simulink model "TemplateNIPID"  (Simulink 7.3)
settings: Solver=ode5  StartTime=0.0  StopTime=inf  FixedStep=0.1  RelTol=1e-3
undefined symbols (not defined in the file): eta1_0_real, v1_0_real, velocitySatValues1
libraries: simulink x41, dspmtrx3 x16, marine_gnc x6, dspindex x5, simulink_extras x1, dspinverses x1
(part 3 of 4)

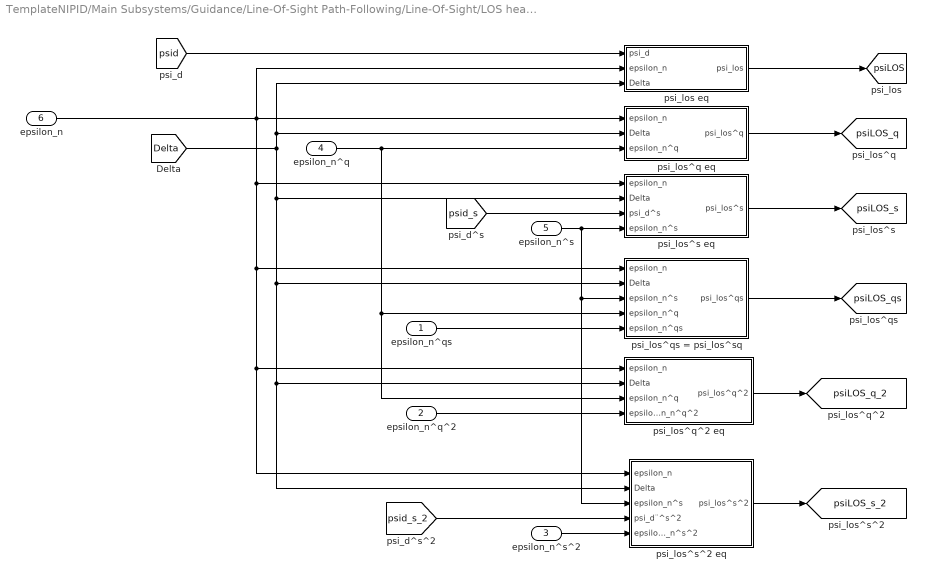
== system TemplateNIPID/Main Subsystems/Guidance/Line-Of-Sight Path-Following/Line-Of-Sight/LOS heading ==
  epsilon_n^qs : Inport
  epsilon_n^q^2 : Inport  Port=2
  epsilon_n^s^2 : Inport  Port=3
  epsilon_n^q : Inport  Port=4
  epsilon_n^s : Inport  Port=5
  epsilon_n : Inport  Port=6
  psi_los eq : Subsystem
  psi_los^q eq : Subsystem
  psi_los^q^2 eq : Subsystem
  psi_los^qs = psi_los^sq : Subsystem
  psi_los^s eq : Subsystem
  psi_los^s^2 eq : Subsystem
  tag scope: psiLOS=global, psiLOS_q=global, psiLOS_q_2=global, psiLOS_qs=global, psiLOS_s=global, psiLOS_s_2=global
  wires:
  psi_los^s^2 eq/1(psi_los^s^2) -> [psiLOS_s_2]
  epsilon_n^s^2/1 -> psi_los^s^2 eq/5(epsilon_n^s^2)
  [psid_s_2] -> psi_los^s^2 eq/4(psi_d¨^s^2)
  epsilon_n^q^2/1 -> psi_los^q^2 eq/4(epsilon_n^q^2)
  psi_los^q^2 eq/1(psi_los^q^2) -> [psiLOS_q_2]
  epsilon_n^qs/1 -> psi_los^qs = psi_los^sq/5(epsilon_n^qs)
  epsilon_n^s/1 -> psi_los^s eq/4(epsilon_n^s), psi_los^s^2 eq/3(epsilon_n^s), psi_los^qs = psi_los^sq/3(epsilon_n^s)
  psi_los^qs = psi_los^sq/1(psi_los^qs) -> [psiLOS_qs]
  [psid_s] -> psi_los^s eq/3(psi_d^s)
  psi_los^s eq/1(psi_los^s) -> [psiLOS_s]
  psi_los^q eq/1(psi_los^q) -> [psiLOS_q]
  epsilon_n^q/1 -> psi_los^q eq/3(epsilon_n^q), psi_los^q^2 eq/3(epsilon_n^q), psi_los^qs = psi_los^sq/4(epsilon_n^q)
  [Delta] -> psi_los^q eq/2(Delta), psi_los^s eq/2(Delta), psi_los^qs = psi_los^sq/2(Delta), psi_los^s^2 eq/2(Delta), psi_los^q^2 eq/2(Delta), psi_los eq/3(Delta)
  epsilon_n/1 -> psi_los^q eq/1(epsilon_n), psi_los^s eq/1(epsilon_n), psi_los^qs = psi_los^sq/1(epsilon_n), psi_los^s^2 eq/1(epsilon_n), psi_los^q^2 eq/1(epsilon_n), psi_los eq/2(epsilon_n)
  [psid] -> psi_los eq/1(psi_d)
  psi_los eq/1(psi_los) -> [psiLOS]

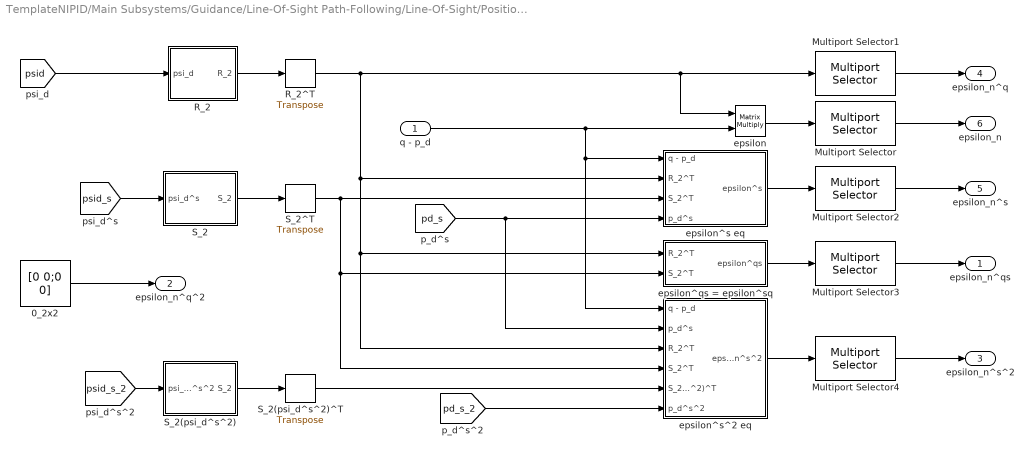
== system TemplateNIPID/Main Subsystems/Guidance/Line-Of-Sight Path-Following/Line-Of-Sight/Position error signals ==
  q - p_d : Inport  OutDataType=fixdt(1, 16)  OutScaling=2^0
  0_2x2 : Constant  Value=[0 0;0 0]  OutDataType=fixdt(1, 16)  OutScaling=2^0
  Multiport Selector{,1..4} (5 alike) : dspindex/Multiport Selector  rowsOrCols=Rows  idxCellArray={2}  idxErrMode=Clip Index
  R_2 : Subsystem  TreatAsAtomicUnit=on
      settings: MinAlgLoopOccurrences=on
  R_2^T : dspmtrx3/Transpose  SystemSampleTime=-1  Hermitian=off  overflowFlag=off
  S_2 : Subsystem  TreatAsAtomicUnit=on
      settings: MinAlgLoopOccurrences=on
  S_2(psi_d^s^2) : Subsystem  TreatAsAtomicUnit=on
      settings: MinAlgLoopOccurrences=on
  S_2(psi_d^s^2)^T : dspmtrx3/Transpose  SystemSampleTime=-1  Hermitian=off  overflowFlag=off
  S_2^T : dspmtrx3/Transpose  SystemSampleTime=-1  Hermitian=off  overflowFlag=off
  epsilon : Product  Multiplication=Matrix(*)  OutDataType=fixdt(1, 16)  OutScaling=2^0  RndMeth=Zero
  epsilon^qs = epsilon^sq : Subsystem
  epsilon^s eq : Subsystem
  epsilon^s^2 eq : Subsystem
  epsilon_n^qs : Outport
  epsilon_n^q^2 : Outport  Port=2
  epsilon_n^s^2 : Outport  Port=3
  epsilon_n^q : Outport  Port=4
  epsilon_n^s : Outport  Port=5
  epsilon_n : Outport  Port=6
  wires:
  Multiport Selector1/1 -> epsilon_n^q/1
  [pd_s_2] -> epsilon^s^2 eq/6(p_d^s^2)
  S_2(psi_d^s^2)^T/1 -> epsilon^s^2 eq/5(S_2(psi_d^s^2)^T)
  Multiport Selector4/1 -> epsilon_n^s^2/1
  epsilon^s^2 eq/1(epsilon^s^2) -> Multiport Selector4/1
  S_2(psi_d^s^2)/1(S_2) -> S_2(psi_d^s^2)^T/1
  Multiport Selector3/1 -> epsilon_n^qs/1
  Multiport Selector2/1 -> epsilon_n^s/1
  Multiport Selector/1 -> epsilon_n/1
  epsilon/1 -> Multiport Selector/1
  0_2x2/1 -> epsilon_n^q^2/1
  epsilon^qs = epsilon^sq/1(epsilon^qs) -> Multiport Selector3/1
  S_2^T/1 -> epsilon^s^2 eq/4(S_2^T), epsilon^qs = epsilon^sq/2(S_2^T), epsilon^s eq/3(S_2^T)
  epsilon^s eq/1(epsilon^s) -> Multiport Selector2/1
  [pd_s] -> epsilon^s^2 eq/2(p_d^s), epsilon^s eq/4(p_d^s)
  S_2/1(S_2) -> S_2^T/1
  q - p_d/1 -> epsilon^s^2 eq/1(q - p_d), epsilon^s eq/1(q - p_d), epsilon/2
  R_2^T/1 -> epsilon^s^2 eq/3(R_2^T), epsilon^qs = epsilon^sq/1(R_2^T), epsilon^s eq/2(R_2^T), Multiport Selector1/1, epsilon/1
  [psid] -> R_2/1(psi_d)
  R_2/1(R_2) -> R_2^T/1
  [psid_s] -> S_2/1(psi_d^s)
  [psid_s_2] -> S_2(psi_d^s^2)/1(psi_d^s^2)

== system TemplateNIPID/Main Subsystems/Guidance/Line-Of-Sight Path-Following/Line-Of-Sight/Virtual Vessel ==
  0_2x1 : Constant  Value=[0;0]  VectorParams1D=off  OutDataType=fixdt(1, 16)  OutScaling=2^0
  I : dspmtrx3/Constant Diagonal Matrix  SystemSampleTime=-1  q=[1 1]  frame=off  dataType=Inherit from 'Constant(s) along diagonal'  isSigned=on  wordLen=16  udDataType=sfix(16)  fracBitsMode=Best precision  numFracBits=15
  Matrix Concatenate : Concatenate  Mode=Multidimensional array
  Vector Concatenate : Concatenate  Mode=Vector
  Vector Concatenate1 : Concatenate  Mode=Vector
  tag scope: chi=global, chi_q=global, chi_s=global
  wires:
  0_2x1/1 -> Vector Concatenate1/1
  Vector Concatenate1/1 -> [chi_s]
  Matrix Concatenate/1 -> [chi_q]
  [psiLOS_q] -> Matrix Concatenate/2
  I/1 -> Matrix Concatenate/1
  Vector Concatenate/1 -> [chi]
  [psiLOS] -> Vector Concatenate/2
  [q] -> Vector Concatenate/1
  [psiLOS_s] -> Vector Concatenate1/2

== system TemplateNIPID/Main Subsystems/Guidance/Line-Of-Sight Path-Following/Path/Ellipse path ==
  p_d eq : Subsystem
  p_d^s eq : Subsystem
  p_d^s^2 eq : Subsystem
  p_d^s^3 eq : Subsystem
  |p_d^s| eq : Subsystem
  tag scope: pdEllipse=global, pd_sEllipse=global, pd_s_2Ellipse=global, pd_s_3Ellipse=global, pd_sabsEllipse=global
  wires:
  p_d^s eq/1(p_d^s) -> [pd_sEllipse], |p_d^s| eq/1(p_d^s)
  [s] -> p_d eq/1(s), p_d^s eq/1(s), p_d^s^2 eq/1(s), p_d^s^3 eq/1(s)
  [rx] -> p_d eq/2(r_x), p_d^s eq/2(r_x), p_d^s^2 eq/2(r_x), p_d^s^3 eq/2(r_x)
  [ry] -> p_d eq/3(r_y), p_d^s eq/3(r_y), p_d^s^2 eq/3(r_y), p_d^s^3 eq/3(r_y)
  [x0] -> p_d eq/4(origo_x)
  [y0] -> p_d eq/5(origo_y)
  [k] -> p_d eq/6(k), p_d^s eq/4(k), p_d^s^2 eq/4(k), p_d^s^3 eq/4(k)
  p_d eq/1(p_d) -> [pdEllipse]
  |p_d^s| eq/1(|p_d^s|) -> [pd_sabsEllipse]
  p_d^s^2 eq/1(p_d^s^2) -> [pd_s_2Ellipse]
  p_d^s^3 eq/1(p_d^s^3) -> [pd_s_3Ellipse]

== system TemplateNIPID/Main Subsystems/Guidance/Line-Of-Sight Path-Following/Path/Path Switch workaround + limiter ==
  note: Path Selector == 1: Linear path
      | Path Selector == 0: Ellipse path
  Limiter : Subsystem
  Rounding Function : Rounding
  Saturation : Saturate  UpperLimit=1  LowerLimit=0  OutDataType=fixdt(1, 16)  OutScaling=2^0
  p_d selcetor : Subsystem
  p_d^s selcetor : Subsystem
  p_d^s^2 selcetor : Subsystem
  p_d^s^3 selcetor : Subsystem
  p_d^s^3 selcetor1 : Subsystem
  tag scope: pd=global, pd_s=global, pd_s_2=global, pd_s_3=global, pd_sabs=global
  wires:
  [pathSelector] -> Saturation/1  "chosen path"
  p_d selcetor/1(p_d) -> Limiter/1(p_d)
  Limiter/1(sat_p_d) -> [pd]
  p_d^s selcetor/1(p_d^s) -> [pd_s]
  p_d^s^2 selcetor/1(p_d^s^2) -> [pd_s_2]
  p_d^s^3 selcetor/1(p_d^s^3) -> [pd_s_3]
  p_d^s^3 selcetor1/1(|p_d^s|) -> [pd_sabs]
  Rounding Function/1 -> p_d selcetor/1(Path Selector), p_d^s selcetor/1(Path Selector), p_d^s^2 selcetor/1(Path Selector), p_d^s^3 selcetor/1(Path Selector), p_d^s^3 selcetor1/1(Path Selector)
  Saturation/1 -> Rounding Function/1

== system TemplateNIPID/Main Subsystems/Guidance/Line-Of-Sight Path-Following/Path/Straight path ==
  0_2x1 : Constant  Value=[0;0]  VectorParams1D=off  OutDataType=fixdt(1, 16)  OutScaling=2^0
  p_d eq : Subsystem
  p_d^s eq : Subsystem
  |p_d^s| eq : Subsystem
  tag scope: pdLinear=global, pd_sLinear=global, pd_s_2Linear=global, pd_s_3Linear=global, pd_sabsLinear=global
  wires:
  p_d eq/1(p_d) -> [pdLinear]
  0_2x1/1 -> [pd_s_2Linear], [pd_s_3Linear]
  [y2] -> p_d eq/5(y_2), p_d^s eq/4(y_2)
  [x2] -> p_d eq/4(x_2), p_d^s eq/3(x_2)
  [y1] -> p_d eq/3(y_1), p_d^s eq/2(y_1)
  [x1] -> p_d eq/2(x_1), p_d^s eq/1(x_1)
  [s] -> p_d eq/1(s)
  |p_d^s| eq/1(|p_d^s|) -> [pd_sabsLinear]
  p_d^s eq/1(p_d^s) -> |p_d^s| eq/1(p_d^s), [pd_sLinear]

== system TemplateNIPID/Main Subsystems/Guidance/Line-Of-Sight Path-Following/Speed assigment/v_s eq ==
  |p_d^s| : Inport
  u_d : Inport  Port=2
  Divide : Product  Inputs=*/  OutDataType=fixdt(1, 16)  OutScaling=2^-10
  v_s : Outport
  wires:
  |p_d^s|/1 -> Divide/2
  u_d/1 -> Divide/1
  Divide/1 -> v_s/1

== system TemplateNIPID/Main Subsystems/Guidance/Line-Of-Sight Path-Following/Speed assigment/v_s^s eq ==
  |p_d^s| : Inport
  u_d : Inport  Port=2
  p_d^s : Inport  Port=3
  p_d^s^2 : Inport  Port=4
  Constant : Constant  Value=3  OutDataType=fixdt(1, 16)  OutScaling=2^0
  Divide : Product  Inputs=*/  OutDataType=fixdt(1, 16)  OutScaling=2^-10
  Gain : Gain  Gain=-1  ParameterDataType=fixdt(1, 16)  ParameterScaling=2^0  OutDataType=fixdt(1, 16)  OutScaling=2^0
  Product : Product  OutDataType=fixdt(1, 16)  OutScaling=2^0  RndMeth=Zero
  Product1 : Product  Multiplication=Matrix(*)  OutDataType=fixdt(1, 16)  OutScaling=2^0  RndMeth=Zero
  p_d^s^T : dspmtrx3/Transpose  SystemSampleTime=-1  Hermitian=off  overflowFlag=off
  |p_d^s|^3 : Math  Operator=pow  OutDataType=fixdt(1, 16)  OutScaling=2^0  SaturateOnIntegerOverflow=on
  v_s^s : Outport
  wires:
  Gain/1 -> v_s^s/1
  u_d/1 -> Product/2
  Divide/1 -> Product/1
  |p_d^s|^3/1 -> Divide/2
  Product1/1 -> Divide/1
  Constant/1 -> |p_d^s|^3/2
  |p_d^s|/1 -> |p_d^s|^3/1
  p_d^s^2/1 -> Product1/2
  p_d^s^T/1 -> Product1/1
  p_d^s/1 -> p_d^s^T/1
  Product/1 -> Gain/1

== system TemplateNIPID/Main Subsystems/Guidance/Line-Of-Sight Path-Following/Speed assigment/v_s^t eq ==
  |p_d^s| : Inport
  u_d^t : Inport  Port=2
  Divide : Product  Inputs=*/  OutDataType=fixdt(1, 16)  OutScaling=2^-10
  v_s^t : Outport
  wires:
  |p_d^s|/1 -> Divide/2
  u_d^t/1 -> Divide/1
  Divide/1 -> v_s^t/1

== system TemplateNIPID/Main Subsystems/Naviagation/Input from SIT/u_act to tau/u_act to f_act ==
  u_act : Inport
  Demux : Demux  Outputs=5
  Mux : Mux  Inputs=5
  u_1 to f_1 VSP speed 0.3 : Subsystem
  u_2 to f_2 VSP speed 0.3 : Subsystem
  u_3 to f_3 VSP speed 0.3 : Subsystem
  u_4 to f_4 VSP speed 0.3 : Subsystem
  u_5 to f_5 BT power 0.4 : Subsystem
  f_act : Outport
  wires:
  Demux/2 -> u_2 to f_2 VSP speed 0.3/1(u_2)
  u_act/1 -> Demux/1
  Mux/1 -> f_act/1
  Demux/1 -> u_1 to f_1 VSP speed 0.3/1(u_1)
  Demux/3 -> u_3 to f_3 VSP speed 0.3/1(u_3)
  Demux/4 -> u_4 to f_4 VSP speed 0.3/1(u_4)
  Demux/5 -> u_5 to f_5 BT power 0.4/1(u_5)
  u_1 to f_1 VSP speed 0.3/1(f_1) -> Mux/1
  u_2 to f_2 VSP speed 0.3/1(f_2) -> Mux/2
  u_3 to f_3 VSP speed 0.3/1(f_3) -> Mux/3
  u_4 to f_4 VSP speed 0.3/1(f_4) -> Mux/4
  u_5 to f_5 BT power 0.4/1(f_5) -> Mux/5

== system TemplateNIPID/Main Subsystems/Plant/Linear Simulator/Linear Vessel Dynamics/R(psi) ==
  psi : Inport
  Mux : Mux  Inputs=9
  R(psi) : Reshape  OutputDimensionality=Customize  OutputDimensions=[3,3]
  R11 : Fcn  Expr=cos(u(1))
  R12 : Fcn  Expr=-1*sin(u(1))
  R{13,23,31..32} (4 alike) : Constant  Value=0
  R21 : Fcn  Expr=sin(u(1))
  R22 : Fcn  Expr=cos(u(1))
  R33 : Constant
  R : Outport
  wires:
  R(psi)/1 -> R/1
  Mux/1 -> R(psi)/1
  psi/1 -> R11/1, R21/1, R12/1, R22/1
  R11/1 -> Mux/1
  R21/1 -> Mux/2
  R31/1 -> Mux/3
  R12/1 -> Mux/4
  R22/1 -> Mux/5
  R32/1 -> Mux/6
  R13/1 -> Mux/7
  R33/1 -> Mux/9
  R23/1 -> Mux/8

== system TemplateNIPID/Main Subsystems/Control/Nonlinear PID/Control law/tau_FF/S(r)^T ==
  Mux : Mux  Inputs=9
  R31 : Constant  Value=0
  S(r) : Reshape  OutputDimensionality=Customize  OutputDimensions=[3,3]
  S{11,13,22..23,32} (5 alike) : Constant  Value=0
  S12 : Gain  ParameterDataType=fixdt(1, 16)  ParameterScaling=2^0  OutDataType=fixdt(1, 16)  OutScaling=2^0
  S33 : Constant
  S^T : dspmtrx3/Transpose  SystemSampleTime=-1  Hermitian=off  overflowFlag=off
  r : Selector  InputPortWidth=3  IndexOptions=Index vector (dialog)  Indices=[3]  OutputSizes=1
  S(r)^T : Outport
  wires:
  S(r)/1 -> S^T/1
  Mux/1 -> S(r)/1
  R31/1 -> Mux/3
  S12/1 -> Mux/4
  S22/1 -> Mux/5
  S32/1 -> Mux/6
  S13/1 -> Mux/7
  S33/1 -> Mux/9
  S23/1 -> Mux/8
  S11/1 -> Mux/1
  r/1 -> Mux/2, S12/1
  [nu] -> r/1
  S^T/1 -> S(r)^T/1

== system TemplateNIPID/Main Subsystems/Control/Nonlinear PID/e_1/Heading to -pi/pi/rad to [-pi pi] ==
  rad : Inport  OutDataType=sfix(16)  OutScaling=2^0
  Constant : Constant  Value=2*pi  OutDataType=sfix(16)  OutScaling=2^0
  Gain : Gain  Gain=pi  ParameterDataType=sfix(16)  ParameterScaling=2^0  OutDataType=sfix(16)  OutScaling=2^0  SaturateOnIntegerOverflow=on  OutDataTypeStr=Inherit: Same as input  ParamDataTypeStr=Inherit: Same as input
  Math Function : Math  Operator=rem  OutDataType=sfix(16)  OutScaling=2^0  SaturateOnIntegerOverflow=on
  Saturation : Saturate  UpperLimit=1e10  LowerLimit=-1e10
  Sign : Signum
  Sum : Sum  Inputs=|+-  OutDataType=sfix(16)  OutScaling=2^0  SaturateOnIntegerOverflow=on
  Sum1 : Sum  Inputs=|++  OutDataType=sfix(16)  OutScaling=2^0  SaturateOnIntegerOverflow=on
  "[-pi pi]" : Outport  OutDataType=sfix(16)  OutScaling=2^0
  wires:
  Sum/1 -> "[-pi pi]"/1
  Math Function/1 -> Sum/1
  Constant/1 -> Math Function/2
  Sum1/1 -> Math Function/1
  Gain/1 -> Sum1/2, Sum/2
  Sign/1 -> Gain/1
  rad/1 -> Saturation/1
  Saturation/1 -> Sign/1, Sum1/1

== system TemplateNIPID/Main Subsystems/Control/Nonlinear PID/e_1/Heading to -pi/pi1/rad to [-pi pi] ==
  rad : Inport  OutDataType=sfix(16)  OutScaling=2^0
  Constant : Constant  Value=2*pi  OutDataType=sfix(16)  OutScaling=2^0
  Gain : Gain  Gain=pi  ParameterDataType=sfix(16)  ParameterScaling=2^0  OutDataType=sfix(16)  OutScaling=2^0  SaturateOnIntegerOverflow=on  OutDataTypeStr=Inherit: Same as input  ParamDataTypeStr=Inherit: Same as input
  Math Function : Math  Operator=rem  OutDataType=sfix(16)  OutScaling=2^0  SaturateOnIntegerOverflow=on
  Saturation : Saturate  UpperLimit=1e10  LowerLimit=-1e10
  Sign : Signum
  Sum : Sum  Inputs=|+-  OutDataType=sfix(16)  OutScaling=2^0  SaturateOnIntegerOverflow=on
  Sum1 : Sum  Inputs=|++  OutDataType=sfix(16)  OutScaling=2^0  SaturateOnIntegerOverflow=on
  "[-pi pi]" : Outport  OutDataType=sfix(16)  OutScaling=2^0
  wires:
  Sum/1 -> "[-pi pi]"/1
  Math Function/1 -> Sum/1
  Constant/1 -> Math Function/2
  Sum1/1 -> Math Function/1
  Gain/1 -> Sum1/2, Sum/2
  Sign/1 -> Gain/1
  rad/1 -> Saturation/1
  Saturation/1 -> Sign/1, Sum1/1

== system TemplateNIPID/Main Subsystems/Control/PS3 u input control/u_act to tau/u_act to f_act/u_1 to f_1 VSP speed 0.3 ==
  note: Table valid for VSP speed == 0.30
  u_1 : Inport
  u_1 to f_1 : Lookup  InputValues=[-1.0000 -0.9500 -0.9000 -0.8500 -0.8000 -0.7500 -0.7000 -0.6500 -0.6000 -0.5500 -0.5000 -0.4500 -0.4000 -0.3500 -0.3000 -0.2500 -0.2000 -0.1500 -0.1000 -0.0500 0 0.0500 0.1000 0.1500 0.2000 0.2500 0.3000 0.3500 0.4000 0.4500 0.5000 0.5500 0.6000 0.6500 0.7000 0.7500 0.8000 0.8500 0.9000]  Table=[-0.6829 -0.6369 -0.5785 -0.5165 -0.4456 -0.3725 -0.3308 -0.2827 -0.2277 -0.1517 -0.1240 -0.0769 -0.0238 0.0039 0.0377 0.0635 0.1051 0.1196 0.1412 0.1721 0.1754 0.1774 0.2104 0.2200 0.2266 0.2673 0.3025 0.3486 0.3896 0.4252 0.4782 0.5164 0.5695 0.6195 0.6723 0.7449 0.7836 0.8414 0.8987 ]  LookUpMeth=Interpolation-Use End Values  OutDataType=fixdt(1, 16)  OutScaling=2^0
  f_1 : Outport
  wires:
  u_1/1 -> u_1 to f_1/1
  u_1 to f_1/1 -> f_1/1

== system TemplateNIPID/Main Subsystems/Control/PS3 u input control/u_act to tau/u_act to f_act/u_2 to f_2 VSP speed 0.3 ==
  note: Switching to the lookup table giving the closes value
  note: workaround setup
  note: Tables valid for VSP speed == 0.30
  u_2 : Inport
  Gain1 : Gain  Gain=3  ParameterDataType=fixdt(1, 16)  ParameterScaling=2^0  OutDataType=fixdt(1, 16)  OutScaling=2^0
  If < 0.00391 : simulink/Logic and Bit Operations/Compare To Constant  SystemSampleTime=-1  relop=<  const=-0.5  LogicOutDataTypeMode=uint8
  If < 0.06731 : simulink/Logic and Bit Operations/Compare To Constant  SystemSampleTime=-1  relop=<  const=-0.1  LogicOutDataTypeMode=uint8
  If >= 0.00391 : simulink/Logic and Bit Operations/Compare To Constant  SystemSampleTime=-1  relop=>=  const=-0.5  LogicOutDataTypeMode=uint8
  If >= 0.06731 : simulink/Logic and Bit Operations/Compare To Constant  SystemSampleTime=-1  relop=>=  const=-0.1  LogicOutDataTypeMode=uint8
  Logical Operator : Logic  AllPortsSameDT=off  OutDataTypeMode=boolean  LogicDataType=fixdt(0, 8)  OutDataTypeStr=boolean
  Multiport Switch : MultiPortSwitch  OutDataType=fixdt(1, 16)  OutScaling=2^0
  Sum : Sum  Inputs=+++  OutDataType=fixdt(1, 16)  OutScaling=2^0
  Sum1 : Sum  Inputs=|++  OutDataType=fixdt(1, 16)  OutScaling=2^0
  u_2 < -0.1 && u_2 >= -0.2 : Lookup  InputValues=|  Table=|  LookUpMeth=Interpolation-Use End Values  OutDataType=fixdt(1, 16)  OutScaling=2^0
      InputValues=|
      | [-0.2000
      |    -0.1500
      |    -0.1000]
      Table=|
      | [-0.0105
      |     0.0226
      |     0.0673]
  u_2 < -0.5 : Lookup  InputValues=|  Table=|  LookUpMeth=Interpolation-Use End Values  OutDataType=fixdt(1, 16)  OutScaling=2^0
      InputValues=|
      | [-1.0000
      |    -0.9500
      |    -0.9000
      |    -0.8500
      |    -0.8000
      |    -0.7500
      |    -0.7000
      |    -0.6500
      |    -0.6000
      |    -0.5500
      |    -0.5000]
      Table=|
      | [-0.2704
      |    -0.2259
      |    -0.1903
      |    -0.1697
      |    -0.1518
      |    -0.1234
      |    -0.0994
      |    -0.0817
      |    -0.0612
      |    -0.0123
      |     0.0039]
  u_2 => 0 : Lookup  InputValues=|  Table=|  LookUpMeth=Interpolation-Use End Values  OutDataType=fixdt(1, 16)  OutScaling=2^0
      InputValues=|
      | [0
      |     0.0500
      |     0.1000
      |     0.1500
      |     0.2000
      |     0.2500
      |     0.3000
      |     0.3500
      |     0.4000
      |     0.4500
      |     0.5000
      |     0.5500
      |     0.6000
      |     0.6500
      |     0.7000
      |     0.7500
      |     0.8000
      |     0.8500]
      Table=|
      | [0.0872
      |     0.0930
      |     0.1182
      |     0.1412
      |     0.1892
      |     0.2146
      |     0.2678
      |     0.3096
      |     0.3551
      |     0.4013
      |     0.4566
      |     0.5051
      |     0.5477
      |     0.6060
      |     0.6703
      |     0.7437
      |     0.7604
      |     0.7634]
  f_2 : Outport
  wires:
  Multiport Switch/1 -> f_2/1
  Sum/1 -> Multiport Switch/1
  If >= 0.06731/1 -> Gain1/1
  If < 0.00391/1 -> Sum/1
  u_2/1 -> u_2 < -0.5/1, If >= 0.06731/1, If < 0.00391/1, If >= 0.00391/1, If < 0.06731/1, u_2 => 0/1, u_2 < -0.1 && u_2 >= -0.2/1
  u_2 < -0.5/1 -> Multiport Switch/2
  u_2 => 0/1 -> Multiport Switch/4
  u_2 < -0.1 && u_2 >= -0.2/1 -> Multiport Switch/3
  If < 0.06731/1 -> Logical Operator/2
  If >= 0.00391/1 -> Logical Operator/1
  Gain1/1 -> Sum/3
  Sum1/1 -> Sum/2
  Logical Operator/1 -> Sum1/1, Sum1/2

== system TemplateNIPID/Main Subsystems/Control/PS3 u input control/u_act to tau/u_act to f_act/u_3 to f_3 VSP speed 0.3 ==
  note: Table valid for VSP speed == 0.30
  u_3 : Inport
  u_3 to f_3 : Lookup  InputValues=[-1.0000,-0.9500,-0.9000,-0.8500,-0.8000,-0.7500,-0.7000,-0.6500,-0.6000,-0.5500,-0.5000,-0.4500,-0.4000,-0.3500,-0.3000,-0.2000,-0.1500,-0.1000,-0.0500,0,0.0500,0.1000,0.1500,0.2000,0.2500,0.3000,0.3500,0.4000,0.4500,0.5000,0.5500,0.6000,0.6500,0.7000,0.7500,0.8000,0.8500,0.9500,1.0000]  Table=[-0.5408,-0.5036,-0.4487,-0.3802,-0.3147,-0.2525,-0.2338,-0.1568,-0.1034,-0.0647,-0.0054,0.0221,0.0572,0.0747,0.0991,0.1258,0.1385,0.1447,0.1539,0.1625,0.1712,0.1976,0.2258,0.2443,0.3058,0.3460,0.3989,0.4342,0.4932,0.5524,0.5814,0.6394,0.6851,0.7496,0.8081,0.8382,0.8665,0.8767,0.8885]  LookUpMeth=Interpolation-Use End Values  OutDataType=fixdt(1, 16)  OutScaling=2^0
  f_3 : Outport
  wires:
  u_3/1 -> u_3 to f_3/1
  u_3 to f_3/1 -> f_3/1

== system TemplateNIPID/Main Subsystems/Control/PS3 u input control/u_act to tau/u_act to f_act/u_4 to f_4 VSP speed 0.3 ==
  note: Tables valid for VSP speed == 0.30
  u_4 : Inport
  Gain : Gain  Gain=2  ParameterDataType=fixdt(1, 16)  ParameterScaling=2^0  OutDataType=fixdt(1, 16)  OutScaling=2^0
  If < 0.0451 : simulink/Logic and Bit Operations/Compare To Constant  SystemSampleTime=-1  relop=<  const=-0.1  LogicOutDataTypeMode=uint8
  If >= 0.0451 : simulink/Logic and Bit Operations/Compare To Constant  SystemSampleTime=-1  relop=>=  const=-0.1  LogicOutDataTypeMode=uint8
  Multiport Switch : MultiPortSwitch  Inputs=2  OutDataType=fixdt(1, 16)  OutScaling=2^0
  Sum : Sum  Inputs=+|+  OutDataType=fixdt(1, 16)  OutScaling=2^0
  u_4 < -0.1 : Lookup  InputValues=|  Table=|  LookUpMeth=Interpolation-Use End Values  OutDataType=fixdt(1, 16)  OutScaling=2^0
      InputValues=|
      | [-0.8000
      |    -0.7500
      |    -0.7000
      |    -0.6500
      |    -0.6000
      |    -0.5500
      |    -0.5000
      |    -0.4500
      |    -0.4000
      |    -0.3500
      |    -0.3000
      |    -0.2500
      |    -0.2000
      |    -0.1500
      |    -0.1000]
      Table=|
      | [-0.5212
      |    -0.5163
      |    -0.4943
      |    -0.4390
      |    -0.3803
      |    -0.3603
      |    -0.3132
      |    -0.2567
      |    -0.2102
      |    -0.1609
      |    -0.1267
      |    -0.0819
      |    -0.0554
      |     0.0099
      |     0.0450]
  u_4 >= -0.1 : Lookup  InputValues=|  Table=|  LookUpMeth=Interpolation-Use End Values  OutDataType=fixdt(1, 16)  OutScaling=2^0
      InputValues=|
      | [0.0431
      |     0.0808
      |     0.0867
      |     0.1337
      |     0.1726
      |     0.1963
      |     0.2088
      |     0.2323
      |     0.2969
      |     0.3134
      |     0.3376
      |     0.3743
      |     0.4276]
      Table=|
      | [0.4000
      |     0.4500
      |     0.5000
      |     0.5500
      |     0.6000
      |     0.6500
      |     0.7000
      |     0.7500
      |     0.8000
      |     0.8500
      |     0.9000
      |     0.9500
      |     1.0000]
  f_4 : Outport
  wires:
  Multiport Switch/1 -> f_4/1
  Gain/1 -> Sum/2
  Sum/1 -> Multiport Switch/1
  If >= 0.0451/1 -> Gain/1
  If < 0.0451/1 -> Sum/1
  u_4/1 -> u_4 < -0.1/1, u_4 >= -0.1/1, If >= 0.0451/1, If < 0.0451/1
  u_4 < -0.1/1 -> Multiport Switch/2
  u_4 >= -0.1/1 -> Multiport Switch/3

== system TemplateNIPID/Main Subsystems/Control/PS3 u input control/u_act to tau/u_act to f_act/u_5 to f_5 BT power 0.4 ==
  note: If < 0: control input is 1
      | if = 0 control input is 2
      | if > 0: control input is 3
  note: Check if the input value is less, equal or greater then zero
  note: The mapping is divided into 3 parts:
      | Negative, zero and positive
  u_5 : Inport
  Dead Zone +-0.01 : DeadZone  LowerValue=-0.01  UpperValue=0.01  SaturateOnIntegerOverflow=on
  Gain : Gain  Gain=2  ParameterDataType=fixdt(1, 16)  ParameterScaling=2^0  OutDataType=fixdt(1, 16)  OutScaling=2^0
  Gain1 : Gain  Gain=3  ParameterDataType=fixdt(1, 16)  ParameterScaling=2^0  OutDataType=fixdt(1, 16)  OutScaling=2^0
  If < 0 : simulink/Logic and Bit Operations/Compare To Constant  SystemSampleTime=-1  relop=<  const=0  LogicOutDataTypeMode=uint8
  If > 0 : simulink/Logic and Bit Operations/Compare To Constant  SystemSampleTime=-1  relop=>  const=0  LogicOutDataTypeMode=uint8
  Multiport Switch : MultiPortSwitch  OutDataType=fixdt(1, 16)  OutScaling=2^0
  Sum : Sum  Inputs=+++  OutDataType=fixdt(1, 16)  OutScaling=2^0
  if == 0 : simulink/Logic and Bit Operations/Compare To Zero  SystemSampleTime=-1  relop===  LogicOutDataTypeMode=uint8
  u_5 < 0 : Lookup  InputValues=|  Table=|  LookUpMeth=Interpolation-Use End Values  OutDataType=fixdt(1, 16)  OutScaling=2^0
      InputValues=|
      | [-0.2000
      |    -0.1900
      |    -0.1700
      |    -0.1500
      |    -0.1300
      |    -0.1100
      |    -0.0900
      |    -0.0700
      |    -0.0500
      |    -0.0300]
      Table=|
      | [-1.1653
      |    -1.1010
      |    -0.9810
      |    -0.8576
      |    -0.7363
      |    -0.5877
      |    -0.4265
      |    -0.2640
      |    -0.1099
      |     0.0031]
  u_5 = 0 : Constant  Value=0  OutDataType=fixdt(1, 16)  OutScaling=2^0
  u_5 > 0 : Lookup  InputValues=|  Table=|  LookUpMeth=Interpolation-Use End Values  OutDataType=fixdt(1, 16)  OutScaling=2^0
      InputValues=|
      | [0.0300
      |     0.0500
      |     0.0700
      |     0.0900
      |     0.1100
      |     0.1300
      |     0.1500
      |     0.1700
      |     0.1900
      |     0.2000]
      Table=|
      | [0.0103
      |     0.0743
      |     0.1937
      |     0.3232
      |     0.4342
      |     0.5862
      |     0.7291
      |     0.8697
      |     0.9681
      |     1.0229]
  f_5 : Outport
  wires:
  Dead Zone +-0.01/1 -> If > 0/1, if == 0/1, If < 0/1
  u_5 > 0/1 -> Multiport Switch/4
  u_5 = 0/1 -> Multiport Switch/3
  u_5 < 0/1 -> Multiport Switch/2
  u_5/1 -> Dead Zone +-0.01/1, u_5 > 0/1, u_5 < 0/1
  If < 0/1 -> Sum/1
  if == 0/1 -> Gain/1
  If > 0/1 -> Gain1/1
  Sum/1 -> Multiport Switch/1
  Gain/1 -> Sum/2
  Gain1/1 -> Sum/3
  Multiport Switch/1 -> f_5/1

== system TemplateNIPID/Main Subsystems/Control/Precision control/u_act to tau/u_act to f_act/u_1 to f_1 VSP speed 0.3 ==
  note: Table valid for VSP speed == 0.30
  u_1 : Inport
  u_1 to f_1 : Lookup  InputValues=[-1.0000 -0.9500 -0.9000 -0.8500 -0.8000 -0.7500 -0.7000 -0.6500 -0.6000 -0.5500 -0.5000 -0.4500 -0.4000 -0.3500 -0.3000 -0.2500 -0.2000 -0.1500 -0.1000 -0.0500 0 0.0500 0.1000 0.1500 0.2000 0.2500 0.3000 0.3500 0.4000 0.4500 0.5000 0.5500 0.6000 0.6500 0.7000 0.7500 0.8000 0.8500 0.9000]  Table=[-0.6829 -0.6369 -0.5785 -0.5165 -0.4456 -0.3725 -0.3308 -0.2827 -0.2277 -0.1517 -0.1240 -0.0769 -0.0238 0.0039 0.0377 0.0635 0.1051 0.1196 0.1412 0.1721 0.1754 0.1774 0.2104 0.2200 0.2266 0.2673 0.3025 0.3486 0.3896 0.4252 0.4782 0.5164 0.5695 0.6195 0.6723 0.7449 0.7836 0.8414 0.8987 ]  LookUpMeth=Interpolation-Use End Values  OutDataType=fixdt(1, 16)  OutScaling=2^0
  f_1 : Outport
  wires:
  u_1/1 -> u_1 to f_1/1
  u_1 to f_1/1 -> f_1/1

== system TemplateNIPID/Main Subsystems/Control/Precision control/u_act to tau/u_act to f_act/u_2 to f_2 VSP speed 0.3 ==
  note: Switching to the lookup table giving the closes value
  note: workaround setup
  note: Tables valid for VSP speed == 0.30
  u_2 : Inport
  Gain1 : Gain  Gain=3  ParameterDataType=fixdt(1, 16)  ParameterScaling=2^0  OutDataType=fixdt(1, 16)  OutScaling=2^0
  If < 0.00391 : simulink/Logic and Bit Operations/Compare To Constant  SystemSampleTime=-1  relop=<  const=-0.5  LogicOutDataTypeMode=uint8
  If < 0.06731 : simulink/Logic and Bit Operations/Compare To Constant  SystemSampleTime=-1  relop=<  const=-0.1  LogicOutDataTypeMode=uint8
  If >= 0.00391 : simulink/Logic and Bit Operations/Compare To Constant  SystemSampleTime=-1  relop=>=  const=-0.5  LogicOutDataTypeMode=uint8
  If >= 0.06731 : simulink/Logic and Bit Operations/Compare To Constant  SystemSampleTime=-1  relop=>=  const=-0.1  LogicOutDataTypeMode=uint8
  Logical Operator : Logic  AllPortsSameDT=off  OutDataTypeMode=boolean  LogicDataType=fixdt(0, 8)  OutDataTypeStr=boolean
  Multiport Switch : MultiPortSwitch  OutDataType=fixdt(1, 16)  OutScaling=2^0
  Sum : Sum  Inputs=+++  OutDataType=fixdt(1, 16)  OutScaling=2^0
  Sum1 : Sum  Inputs=|++  OutDataType=fixdt(1, 16)  OutScaling=2^0
  u_2 < -0.1 && u_2 >= -0.2 : Lookup  InputValues=|  Table=|  LookUpMeth=Interpolation-Use End Values  OutDataType=fixdt(1, 16)  OutScaling=2^0
      InputValues=|
      | [-0.2000
      |    -0.1500
      |    -0.1000]
      Table=|
      | [-0.0105
      |     0.0226
      |     0.0673]
  u_2 < -0.5 : Lookup  InputValues=|  Table=|  LookUpMeth=Interpolation-Use End Values  OutDataType=fixdt(1, 16)  OutScaling=2^0
      InputValues=|
      | [-1.0000
      |    -0.9500
      |    -0.9000
      |    -0.8500
      |    -0.8000
      |    -0.7500
      |    -0.7000
      |    -0.6500
      |    -0.6000
      |    -0.5500
      |    -0.5000]
      Table=|
      | [-0.2704
      |    -0.2259
      |    -0.1903
      |    -0.1697
      |    -0.1518
      |    -0.1234
      |    -0.0994
      |    -0.0817
      |    -0.0612
      |    -0.0123
      |     0.0039]
  u_2 => 0 : Lookup  InputValues=|  Table=|  LookUpMeth=Interpolation-Use End Values  OutDataType=fixdt(1, 16)  OutScaling=2^0
      InputValues=|
      | [0
      |     0.0500
      |     0.1000
      |     0.1500
      |     0.2000
      |     0.2500
      |     0.3000
      |     0.3500
      |     0.4000
      |     0.4500
      |     0.5000
      |     0.5500
      |     0.6000
      |     0.6500
      |     0.7000
      |     0.7500
      |     0.8000
      |     0.8500]
      Table=|
      | [0.0872
      |     0.0930
      |     0.1182
      |     0.1412
      |     0.1892
      |     0.2146
      |     0.2678
      |     0.3096
      |     0.3551
      |     0.4013
      |     0.4566
      |     0.5051
      |     0.5477
      |     0.6060
      |     0.6703
      |     0.7437
      |     0.7604
      |     0.7634]
  f_2 : Outport
  wires:
  Multiport Switch/1 -> f_2/1
  Sum/1 -> Multiport Switch/1
  If >= 0.06731/1 -> Gain1/1
  If < 0.00391/1 -> Sum/1
  u_2/1 -> u_2 < -0.5/1, If >= 0.06731/1, If < 0.00391/1, If >= 0.00391/1, If < 0.06731/1, u_2 => 0/1, u_2 < -0.1 && u_2 >= -0.2/1
  u_2 < -0.5/1 -> Multiport Switch/2
  u_2 => 0/1 -> Multiport Switch/4
  u_2 < -0.1 && u_2 >= -0.2/1 -> Multiport Switch/3
  If < 0.06731/1 -> Logical Operator/2
  If >= 0.00391/1 -> Logical Operator/1
  Gain1/1 -> Sum/3
  Sum1/1 -> Sum/2
  Logical Operator/1 -> Sum1/1, Sum1/2

== system TemplateNIPID/Main Subsystems/Control/Precision control/u_act to tau/u_act to f_act/u_3 to f_3 VSP speed 0.3 ==
  note: Table valid for VSP speed == 0.30
  u_3 : Inport
  u_3 to f_3 : Lookup  InputValues=[-1.0000,-0.9500,-0.9000,-0.8500,-0.8000,-0.7500,-0.7000,-0.6500,-0.6000,-0.5500,-0.5000,-0.4500,-0.4000,-0.3500,-0.3000,-0.2000,-0.1500,-0.1000,-0.0500,0,0.0500,0.1000,0.1500,0.2000,0.2500,0.3000,0.3500,0.4000,0.4500,0.5000,0.5500,0.6000,0.6500,0.7000,0.7500,0.8000,0.8500,0.9500,1.0000]  Table=[-0.5408,-0.5036,-0.4487,-0.3802,-0.3147,-0.2525,-0.2338,-0.1568,-0.1034,-0.0647,-0.0054,0.0221,0.0572,0.0747,0.0991,0.1258,0.1385,0.1447,0.1539,0.1625,0.1712,0.1976,0.2258,0.2443,0.3058,0.3460,0.3989,0.4342,0.4932,0.5524,0.5814,0.6394,0.6851,0.7496,0.8081,0.8382,0.8665,0.8767,0.8885]  LookUpMeth=Interpolation-Use End Values  OutDataType=fixdt(1, 16)  OutScaling=2^0
  f_3 : Outport
  wires:
  u_3/1 -> u_3 to f_3/1
  u_3 to f_3/1 -> f_3/1

== system TemplateNIPID/Main Subsystems/Control/Precision control/u_act to tau/u_act to f_act/u_4 to f_4 VSP speed 0.3 ==
  note: Tables valid for VSP speed == 0.30
  u_4 : Inport
  Gain : Gain  Gain=2  ParameterDataType=fixdt(1, 16)  ParameterScaling=2^0  OutDataType=fixdt(1, 16)  OutScaling=2^0
  If < 0.0451 : simulink/Logic and Bit Operations/Compare To Constant  SystemSampleTime=-1  relop=<  const=-0.1  LogicOutDataTypeMode=uint8
  If >= 0.0451 : simulink/Logic and Bit Operations/Compare To Constant  SystemSampleTime=-1  relop=>=  const=-0.1  LogicOutDataTypeMode=uint8
  Multiport Switch : MultiPortSwitch  Inputs=2  OutDataType=fixdt(1, 16)  OutScaling=2^0
  Sum : Sum  Inputs=+|+  OutDataType=fixdt(1, 16)  OutScaling=2^0
  u_4 < -0.1 : Lookup  InputValues=|  Table=|  LookUpMeth=Interpolation-Use End Values  OutDataType=fixdt(1, 16)  OutScaling=2^0
      InputValues=|
      | [-0.8000
      |    -0.7500
      |    -0.7000
      |    -0.6500
      |    -0.6000
      |    -0.5500
      |    -0.5000
      |    -0.4500
      |    -0.4000
      |    -0.3500
      |    -0.3000
      |    -0.2500
      |    -0.2000
      |    -0.1500
      |    -0.1000]
      Table=|
      | [-0.5212
      |    -0.5163
      |    -0.4943
      |    -0.4390
      |    -0.3803
      |    -0.3603
      |    -0.3132
      |    -0.2567
      |    -0.2102
      |    -0.1609
      |    -0.1267
      |    -0.0819
      |    -0.0554
      |     0.0099
      |     0.0450]
  u_4 >= -0.1 : Lookup  InputValues=|  Table=|  LookUpMeth=Interpolation-Use End Values  OutDataType=fixdt(1, 16)  OutScaling=2^0
      InputValues=|
      | [0.0431
      |     0.0808
      |     0.0867
      |     0.1337
      |     0.1726
      |     0.1963
      |     0.2088
      |     0.2323
      |     0.2969
      |     0.3134
      |     0.3376
      |     0.3743
      |     0.4276]
      Table=|
      | [0.4000
      |     0.4500
      |     0.5000
      |     0.5500
      |     0.6000
      |     0.6500
      |     0.7000
      |     0.7500
      |     0.8000
      |     0.8500
      |     0.9000
      |     0.9500
      |     1.0000]
  f_4 : Outport
  wires:
  Multiport Switch/1 -> f_4/1
  Gain/1 -> Sum/2
  Sum/1 -> Multiport Switch/1
  If >= 0.0451/1 -> Gain/1
  If < 0.0451/1 -> Sum/1
  u_4/1 -> u_4 < -0.1/1, u_4 >= -0.1/1, If >= 0.0451/1, If < 0.0451/1
  u_4 < -0.1/1 -> Multiport Switch/2
  u_4 >= -0.1/1 -> Multiport Switch/3

== system TemplateNIPID/Main Subsystems/Control/Precision control/u_act to tau/u_act to f_act/u_5 to f_5 BT power 0.4 ==
  note: If < 0: control input is 1
      | if = 0 control input is 2
      | if > 0: control input is 3
  note: Check if the input value is less, equal or greater then zero
  note: The mapping is divided into 3 parts:
      | Negative, zero and positive
  u_5 : Inport
  Dead Zone +-0.01 : DeadZone  LowerValue=-0.01  UpperValue=0.01  SaturateOnIntegerOverflow=on
  Gain : Gain  Gain=2  ParameterDataType=fixdt(1, 16)  ParameterScaling=2^0  OutDataType=fixdt(1, 16)  OutScaling=2^0
  Gain1 : Gain  Gain=3  ParameterDataType=fixdt(1, 16)  ParameterScaling=2^0  OutDataType=fixdt(1, 16)  OutScaling=2^0
  If < 0 : simulink/Logic and Bit Operations/Compare To Constant  SystemSampleTime=-1  relop=<  const=0  LogicOutDataTypeMode=uint8
  If > 0 : simulink/Logic and Bit Operations/Compare To Constant  SystemSampleTime=-1  relop=>  const=0  LogicOutDataTypeMode=uint8
  Multiport Switch : MultiPortSwitch  OutDataType=fixdt(1, 16)  OutScaling=2^0
  Sum : Sum  Inputs=+++  OutDataType=fixdt(1, 16)  OutScaling=2^0
  if == 0 : simulink/Logic and Bit Operations/Compare To Zero  SystemSampleTime=-1  relop===  LogicOutDataTypeMode=uint8
  u_5 < 0 : Lookup  InputValues=|  Table=|  LookUpMeth=Interpolation-Use End Values  OutDataType=fixdt(1, 16)  OutScaling=2^0
      InputValues=|
      | [-0.2000
      |    -0.1900
      |    -0.1700
      |    -0.1500
      |    -0.1300
      |    -0.1100
      |    -0.0900
      |    -0.0700
      |    -0.0500
      |    -0.0300]
      Table=|
      | [-1.1653
      |    -1.1010
      |    -0.9810
      |    -0.8576
      |    -0.7363
      |    -0.5877
      |    -0.4265
      |    -0.2640
      |    -0.1099
      |     0.0031]
  u_5 = 0 : Constant  Value=0  OutDataType=fixdt(1, 16)  OutScaling=2^0
  u_5 > 0 : Lookup  InputValues=|  Table=|  LookUpMeth=Interpolation-Use End Values  OutDataType=fixdt(1, 16)  OutScaling=2^0
      InputValues=|
      | [0.0300
      |     0.0500
      |     0.0700
      |     0.0900
      |     0.1100
      |     0.1300
      |     0.1500
      |     0.1700
      |     0.1900
      |     0.2000]
      Table=|
      | [0.0103
      |     0.0743
      |     0.1937
      |     0.3232
      |     0.4342
      |     0.5862
      |     0.7291
      |     0.8697
      |     0.9681
      |     1.0229]
  f_5 : Outport
  wires:
  Dead Zone +-0.01/1 -> If > 0/1, if == 0/1, If < 0/1
  u_5 > 0/1 -> Multiport Switch/4
  u_5 = 0/1 -> Multiport Switch/3
  u_5 < 0/1 -> Multiport Switch/2
  u_5/1 -> Dead Zone +-0.01/1, u_5 > 0/1, u_5 < 0/1
  If < 0/1 -> Sum/1
  if == 0/1 -> Gain/1
  If > 0/1 -> Gain1/1
  Sum/1 -> Multiport Switch/1
  Gain/1 -> Sum/2
  Gain1/1 -> Sum/3
  Multiport Switch/1 -> f_5/1

== system TemplateNIPID/Main Subsystems/Control/Thruster allocation/VSP030 BT040/f_act to u_act/f_1 to u_1 VSP speed 0.3 ==
  note: Table valid for VSP speed == 0.30
  f_1 : Inport
  f_1 to u_1 : Lookup  InputValues=[-0.6829 -0.6369 -0.5785 -0.5165 -0.4456 -0.3725 -0.3308 -0.2827 -0.2277 -0.1517 -0.1240 -0.0769 -0.0238 0.0039 0.0377 0.0635 0.1051 0.1196 0.1412 0.1721 0.1754 0.1774 0.2104 0.2200 0.2266 0.2673 0.3025 0.3486 0.3896 0.4252 0.4782 0.5164 0.5695 0.6195 0.6723 0.7449 0.7836 0.8414 0.8987 ]  Table=[-1.0000 -0.9500 -0.9000 -0.8500 -0.8000 -0.7500 -0.7000 -0.6500 -0.6000 -0.5500 -0.5000 -0.4500 -0.4000 -0.3500 -0.3000 -0.2500 -0.2000 -0.1500 -0.1000 -0.0500 0 0.0500 0.1000 0.1500 0.2000 0.2500 0.3000 0.3500 0.4000 0.4500 0.5000 0.5500 0.6000 0.6500 0.7000 0.7500 0.8000 0.8500 0.9000]  LookUpMeth=Interpolation-Use End Values  OutDataType=fixdt(1, 16)  OutScaling=2^0
  u_1 : Outport
  wires:
  f_1 to u_1/1 -> u_1/1
  f_1/1 -> f_1 to u_1/1

== system TemplateNIPID/Main Subsystems/Control/Thruster allocation/VSP030 BT040/f_act to u_act/f_2 to u_2 VSP speed 0.3 ==
  note: Tables valid for VSP speed == 0.30
  note: workaround setup
  note: Switching to the lookup table giving the closes value
  f_2 : Inport
  Gain1 : Gain  Gain=3  ParameterDataType=fixdt(1, 16)  ParameterScaling=2^0  OutDataType=fixdt(1, 16)  OutScaling=2^0
  If < 0.00391 : simulink/Logic and Bit Operations/Compare To Constant  SystemSampleTime=-1  relop=<  const=0.00391  LogicOutDataTypeMode=uint8
  If < 0.06731 : simulink/Logic and Bit Operations/Compare To Constant  SystemSampleTime=-1  relop=<  const=0.06731  LogicOutDataTypeMode=uint8
  If >= 0.00391 : simulink/Logic and Bit Operations/Compare To Constant  SystemSampleTime=-1  relop=>=  const=0.00391  LogicOutDataTypeMode=uint8
  If >= 0.06731 : simulink/Logic and Bit Operations/Compare To Constant  SystemSampleTime=-1  relop=>=  const=0.06731  LogicOutDataTypeMode=uint8
  Logical Operator : Logic  AllPortsSameDT=off  OutDataTypeMode=boolean  LogicDataType=fixdt(0, 8)  OutDataTypeStr=boolean
  Multiport Switch : MultiPortSwitch  OutDataType=fixdt(1, 16)  OutScaling=2^0
  Sum : Sum  Inputs=+++  OutDataType=fixdt(1, 16)  OutScaling=2^0
  Sum1 : Sum  Inputs=|++  OutDataType=fixdt(1, 16)  OutScaling=2^0
  f_2 < 0.00391 : Lookup  InputValues=|  Table=|  LookUpMeth=Interpolation-Use End Values  OutDataType=fixdt(1, 16)  OutScaling=2^0
      InputValues=|
      | [-0.2704
      |    -0.2259
      |    -0.1903
      |    -0.1697
      |    -0.1518
      |    -0.1234
      |    -0.0994
      |    -0.0817
      |    -0.0612
      |    -0.0123
      |     0.0039]
      Table=|
      | [-1.0000
      |    -0.9500
      |    -0.9000
      |    -0.8500
      |    -0.8000
      |    -0.7500
      |    -0.7000
      |    -0.6500
      |    -0.6000
      |    -0.5500
      |    -0.5000]
  f_2 < 0.06731 && f_2 >= 0.00391 : Lookup  InputValues=|  Table=|  LookUpMeth=Interpolation-Use End Values  OutDataType=fixdt(1, 16)  OutScaling=2^0
      InputValues=|
      | [-0.0105
      |     0.0226
      |     0.0673]
      Table=|
      | [-0.2000
      |    -0.1500
      |    -0.1000]
  f_2 => 0.06731 : Lookup  InputValues=|  Table=|  LookUpMeth=Interpolation-Use End Values  OutDataType=fixdt(1, 16)  OutScaling=2^0
      InputValues=|
      | [0.0872
      |     0.0930
      |     0.1182
      |     0.1412
      |     0.1892
      |     0.2146
      |     0.2678
      |     0.3096
      |     0.3551
      |     0.4013
      |     0.4566
      |     0.5051
      |     0.5477
      |     0.6060
      |     0.6703
      |     0.7437
      |     0.7604
      |     0.7634]
      Table=|
      | [0
      |     0.0500
      |     0.1000
      |     0.1500
      |     0.2000
      |     0.2500
      |     0.3000
      |     0.3500
      |     0.4000
      |     0.4500
      |     0.5000
      |     0.5500
      |     0.6000
      |     0.6500
      |     0.7000
      |     0.7500
      |     0.8000
      |     0.8500]
  u_2 : Outport
  wires:
  Logical Operator/1 -> Sum1/2, Sum1/1
  Sum1/1 -> Sum/2
  Gain1/1 -> Sum/3
  If >= 0.00391/1 -> Logical Operator/1
  If < 0.06731/1 -> Logical Operator/2
  f_2 < 0.06731 && f_2 >= 0.00391/1 -> Multiport Switch/3
  f_2 => 0.06731/1 -> Multiport Switch/4
  f_2 < 0.00391/1 -> Multiport Switch/2
  f_2/1 -> f_2 < 0.06731 && f_2 >= 0.00391/1, f_2 => 0.06731/1, If < 0.06731/1, If >= 0.00391/1, If < 0.00391/1, If >= 0.06731/1, f_2 < 0.00391/1
  If < 0.00391/1 -> Sum/1
  If >= 0.06731/1 -> Gain1/1
  Sum/1 -> Multiport Switch/1
  Multiport Switch/1 -> u_2/1

== system TemplateNIPID/Main Subsystems/Control/Thruster allocation/VSP030 BT040/f_act to u_act/f_3 to u_3 VSP speed 0.3 ==
  note: Table valid for VSP speed == 0.30
  f_3 : Inport
  f_3 to u_3 : Lookup  InputValues=[-0.5408,-0.5036,-0.4487,-0.3802,-0.3147,-0.2525,-0.2338,-0.1568,-0.1034,-0.0647,-0.0054,0.0221,0.0572,0.0747,0.0991,0.1258,0.1385,0.1447,0.1539,0.1625,0.1712,0.1976,0.2258,0.2443,0.3058,0.3460,0.3989,0.4342,0.4932,0.5524,0.5814,0.6394,0.6851,0.7496,0.8081,0.8382,0.8665,0.8767,0.8885]  Table=[-1.0000,-0.9500,-0.9000,-0.8500,-0.8000,-0.7500,-0.7000,-0.6500,-0.6000,-0.5500,-0.5000,-0.4500,-0.4000,-0.3500,-0.3000,-0.2000,-0.1500,-0.1000,-0.0500,0,0.0500,0.1000,0.1500,0.2000,0.2500,0.3000,0.3500,0.4000,0.4500,0.5000,0.5500,0.6000,0.6500,0.7000,0.7500,0.8000,0.8500,0.9500,1.0000]  LookUpMeth=Interpolation-Use End Values  OutDataType=fixdt(1, 16)  OutScaling=2^0
  u_3 : Outport
  wires:
  f_3 to u_3/1 -> u_3/1
  f_3/1 -> f_3 to u_3/1

== system TemplateNIPID/Main Subsystems/Control/Thruster allocation/VSP030 BT040/f_act to u_act/f_4 to u_4 VSP speed 0.3 ==
  note: Tables valid for VSP speed == 0.30
  f_4 : Inport
  Gain : Gain  Gain=2  ParameterDataType=fixdt(1, 16)  ParameterScaling=2^0  OutDataType=fixdt(1, 16)  OutScaling=2^0
  If < 0.0451 : simulink/Logic and Bit Operations/Compare To Constant  SystemSampleTime=-1  relop=<  const=.0451  LogicOutDataTypeMode=uint8
  If >= 0.0451 : simulink/Logic and Bit Operations/Compare To Constant  SystemSampleTime=-1  relop=>=  const=0.0451  LogicOutDataTypeMode=uint8
  Multiport Switch : MultiPortSwitch  Inputs=2  OutDataType=fixdt(1, 16)  OutScaling=2^0
  Sum : Sum  Inputs=+|+  OutDataType=fixdt(1, 16)  OutScaling=2^0
  f_4 < 0.0451 : Lookup  InputValues=|  Table=|  LookUpMeth=Interpolation-Use End Values  OutDataType=fixdt(1, 16)  OutScaling=2^0
      InputValues=|
      | [-0.5212
      |    -0.5163
      |    -0.4943
      |    -0.4390
      |    -0.3803
      |    -0.3603
      |    -0.3132
      |    -0.2567
      |    -0.2102
      |    -0.1609
      |    -0.1267
      |    -0.0819
      |    -0.0554
      |     0.0099
      |     0.0450]
      Table=|
      | [-0.8000
      |    -0.7500
      |    -0.7000
      |    -0.6500
      |    -0.6000
      |    -0.5500
      |    -0.5000
      |    -0.4500
      |    -0.4000
      |    -0.3500
      |    -0.3000
      |    -0.2500
      |    -0.2000
      |    -0.1500
      |    -0.1000]
  "f_4 >= 0.0451 " : Lookup  InputValues=|  Table=|  LookUpMeth=Interpolation-Use End Values  OutDataType=fixdt(1, 16)  OutScaling=2^0
      InputValues=|
      | [0.0431
      |     0.0808
      |     0.0867
      |     0.1337
      |     0.1726
      |     0.1963
      |     0.2088
      |     0.2323
      |     0.2969
      |     0.3134
      |     0.3376
      |     0.3743
      |     0.4276]
      Table=|
      | [0.4000
      |     0.4500
      |     0.5000
      |     0.5500
      |     0.6000
      |     0.6500
      |     0.7000
      |     0.7500
      |     0.8000
      |     0.8500
      |     0.9000
      |     0.9500
      |     1.0000]
  u_4 : Outport
  wires:
  "f_4 >= 0.0451 "/1 -> Multiport Switch/3
  f_4 < 0.0451/1 -> Multiport Switch/2
  f_4/1 -> If < 0.0451/1, If >= 0.0451/1, "f_4 >= 0.0451 "/1, f_4 < 0.0451/1
  If < 0.0451/1 -> Sum/1
  If >= 0.0451/1 -> Gain/1
  Sum/1 -> Multiport Switch/1
  Gain/1 -> Sum/2
  Multiport Switch/1 -> u_4/1

== system TemplateNIPID/Main Subsystems/Control/Thruster allocation/VSP030 BT040/f_act to u_act/f_5 to u_5 BT power 0.4 ==
  note: The mapping is divided into 3 parts:
      | Negative, zero and positive
  note: Check if the input value is less, equal or greater then zero
  note: If < 0: control input is 1
      | if = 0 control input is 2
      | if > 0: control input is 3
  f_5 : Inport
  Dead Zone +-0.01 : DeadZone  LowerValue=-0.01  UpperValue=0.01  SaturateOnIntegerOverflow=on
  Gain : Gain  Gain=2  ParameterDataType=fixdt(1, 16)  ParameterScaling=2^0  OutDataType=fixdt(1, 16)  OutScaling=2^0
  Gain1 : Gain  Gain=3  ParameterDataType=fixdt(1, 16)  ParameterScaling=2^0  OutDataType=fixdt(1, 16)  OutScaling=2^0
  If < 0 : simulink/Logic and Bit Operations/Compare To Constant  SystemSampleTime=-1  relop=<  const=0  LogicOutDataTypeMode=uint8
  If > 0 : simulink/Logic and Bit Operations/Compare To Constant  SystemSampleTime=-1  relop=>  const=0  LogicOutDataTypeMode=uint8
  Multiport Switch : MultiPortSwitch  OutDataType=fixdt(1, 16)  OutScaling=2^0
  Sum : Sum  Inputs=+++  OutDataType=fixdt(1, 16)  OutScaling=2^0
  f_5 < 0 : Lookup  InputValues=|  Table=|  LookUpMeth=Interpolation-Use End Values  OutDataType=fixdt(1, 16)  OutScaling=2^0
      InputValues=|
      | [-1.1653
      |    -1.1010
      |    -0.9810
      |    -0.8576
      |    -0.7363
      |    -0.5877
      |    -0.4265
      |    -0.2640
      |    -0.1099
      |     0.0031]
      Table=|
      | [-0.2000
      |    -0.1900
      |    -0.1700
      |    -0.1500
      |    -0.1300
      |    -0.1100
      |    -0.0900
      |    -0.0700
      |    -0.0500
      |    -0.0300]
  f_5 = 0 : Constant  Value=0  OutDataType=fixdt(1, 16)  OutScaling=2^0
  f_5 > 0 : Lookup  InputValues=|  Table=|  LookUpMeth=Interpolation-Use End Values  OutDataType=fixdt(1, 16)  OutScaling=2^0
      InputValues=|
      | [0.0103
      |     0.0743
      |     0.1937
      |     0.3232
      |     0.4342
      |     0.5862
      |     0.7291
      |     0.8697
      |     0.9681
      |     1.0229]
      Table=|
      | [0.0300
      |     0.0500
      |     0.0700
      |     0.0900
      |     0.1100
      |     0.1300
      |     0.1500
      |     0.1700
      |     0.1900
      |     0.2000]
  if == 0 : simulink/Logic and Bit Operations/Compare To Zero  SystemSampleTime=-1  relop===  LogicOutDataTypeMode=uint8
  u_5 : Outport
  wires:
  Multiport Switch/1 -> u_5/1
  Gain1/1 -> Sum/3
  Gain/1 -> Sum/2
  Sum/1 -> Multiport Switch/1
  If > 0/1 -> Gain1/1
  if == 0/1 -> Gain/1
  If < 0/1 -> Sum/1
  f_5/1 -> f_5 < 0/1, f_5 > 0/1, Dead Zone +-0.01/1
  f_5 < 0/1 -> Multiport Switch/2
  f_5 = 0/1 -> Multiport Switch/3
  f_5 > 0/1 -> Multiport Switch/4
  Dead Zone +-0.01/1 -> If < 0/1, if == 0/1, If > 0/1

== system TemplateNIPID/Main Subsystems/Guidance/Line-Of-Sight Path-Following/Heading/psi_d eq/rad to [-pi pi] ==
  rad : Inport  OutDataType=sfix(16)  OutScaling=2^0
  Constant : Constant  Value=2*pi  OutDataType=sfix(16)  OutScaling=2^0
  Gain : Gain  Gain=pi  ParameterDataType=sfix(16)  ParameterScaling=2^0  OutDataType=sfix(16)  OutScaling=2^0  SaturateOnIntegerOverflow=on  OutDataTypeStr=Inherit: Same as input  ParamDataTypeStr=Inherit: Same as input
  Math Function : Math  Operator=rem  OutDataType=sfix(16)  OutScaling=2^0  SaturateOnIntegerOverflow=on
  Saturation : Saturate  UpperLimit=1e10  LowerLimit=-1e10
  Sign : Signum
  Sum : Sum  Inputs=|+-  OutDataType=sfix(16)  OutScaling=2^0  SaturateOnIntegerOverflow=on
  Sum1 : Sum  Inputs=|++  OutDataType=sfix(16)  OutScaling=2^0  SaturateOnIntegerOverflow=on
  "[-pi pi]" : Outport  OutDataType=sfix(16)  OutScaling=2^0
  wires:
  Saturation/1 -> Sum1/1, Sign/1
  rad/1 -> Saturation/1
  Sign/1 -> Gain/1
  Gain/1 -> Sum/2, Sum1/2
  Sum1/1 -> Math Function/1
  Constant/1 -> Math Function/2
  Math Function/1 -> Sum/1
  Sum/1 -> "[-pi pi]"/1

== system TemplateNIPID/Main Subsystems/Guidance/Line-Of-Sight Path-Following/Line-Of-Sight/Dynamic LOS assigment for qdot/f_q eq ==
  psi_los : Inport
  u_d : Inport  Port=2
  Mux : Mux  Inputs=2
  Product : Product  Multiplication=Matrix(*)  OutDataType=fixdt(1, 16)  OutScaling=2^0  RndMeth=Zero
  f_qx : Trigonometry  Operator=cos
  f_qy : Trigonometry
  f_q : Outport
  wires:
  Product/1 -> f_q/1
  u_d/1 -> Product/2
  Mux/1 -> Product/1
  f_qy/1 -> Mux/2
  f_qx/1 -> Mux/1
  psi_los/1 -> f_qy/1, f_qx/1

== system TemplateNIPID/Main Subsystems/Guidance/Line-Of-Sight Path-Following/Line-Of-Sight/Dynamic LOS assigment for qdot/f_q^q eq ==
  psi_los : Inport
  u_d : Inport  Port=2
  psi_los^q : Inport  Port=3
  Gain : Gain  Gain=-1  ParameterDataType=fixdt(1, 16)  ParameterScaling=2^0  OutDataType=fixdt(1, 16)  OutScaling=2^0
  Matrix Concatenate : Concatenate  Mode=Multidimensional array
  Product : Product  OutDataType=fixdt(1, 16)  OutScaling=2^0  RndMeth=Zero
  Product1 : Product  Multiplication=Matrix(*)  OutDataType=fixdt(1, 16)  OutScaling=2^0  RndMeth=Zero
  Product2 : Product  Multiplication=Matrix(*)  OutDataType=fixdt(1, 16)  OutScaling=2^0  RndMeth=Zero
  Trigonometric Function : Trigonometry  Operator=cos
  Trigonometric Function1 : Trigonometry
  "f_q^q " : Outport
  wires:
  Matrix Concatenate/1 -> Product/1
  Product2/1 -> Matrix Concatenate/2
  Product1/1 -> Matrix Concatenate/1
  Trigonometric Function/1 -> Product2/1
  psi_los^q/1 -> Product2/2, Product1/2
  Gain/1 -> Product1/1
  Trigonometric Function1/1 -> Gain/1
  Product/1 -> "f_q^q "/1
  u_d/1 -> Product/2
  psi_los/1 -> Trigonometric Function/1, Trigonometric Function1/1

== system TemplateNIPID/Main Subsystems/Guidance/Line-Of-Sight Path-Following/Line-Of-Sight/Dynamic LOS assigment for qdot/f_q^s eq ==
  psi_los : Inport
  u_d : Inport  Port=2
  psi_los^s : Inport  Port=3
  Gain : Gain  Gain=-1  ParameterDataType=fixdt(1, 16)  ParameterScaling=2^0  OutDataType=fixdt(1, 16)  OutScaling=2^0
  Mux : Mux  Inputs=2
  Product : Product  Multiplication=Matrix(*)  OutDataType=fixdt(1, 16)  OutScaling=2^0  RndMeth=Zero
  Product1 : Product  OutDataType=fixdt(1, 16)  OutScaling=2^0  RndMeth=Zero
  Product2 : Product  OutDataType=fixdt(1, 16)  OutScaling=2^0  RndMeth=Zero
  Trigonometric Function : Trigonometry  Operator=cos
  Trigonometric Function1 : Trigonometry
  f_q^s : Outport
  wires:
  Mux/1 -> Product/1
  Product2/1 -> Mux/2
  Product1/1 -> Mux/1
  Trigonometric Function/1 -> Product2/1
  psi_los^s/1 -> Product2/2, Product1/2
  Gain/1 -> Product1/1
  Trigonometric Function1/1 -> Gain/1
  Product/1 -> f_q^s/1
  u_d/1 -> Product/2
  psi_los/1 -> Trigonometric Function/1, Trigonometric Function1/1
